simulink model "Clock_verif"  (Simulink 7.2)
settings: Solver=ode45  StartTime=0.0  StopTime=10.0  RelTol=1e-3
undefined symbols (not defined in the file): clock_sample
settings Model: Creator=Romain  LastModifiedBy=Romain
settings OptimizationCC: ExpressionDepthLimit=128
settings DebuggingCC: SolverPrmCheckMsg=none  FcnCallInpInsideContextMsg=Enable All  StateNameClashWarn=none  StrictBusMsg=ErrorLevel1
settings CodeAppCC: CustomSymbolStrType=$N$R$M_T
settings GRTTargetCC: TargetFunctionLibrary=C89/C90 (ANSI)

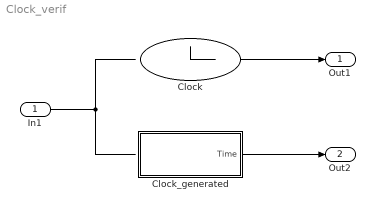
== system Clock_verif ==
  In1 : Inport  OutDataTypeStr=double  DataType=double
  Clock : Clock
  Clock_generated : Subsystem  TreatAsAtomicUnit=on
  Out1 : Outport
  Out2 : Outport  Port=2
  wires:
  In1/1 -> ?
  Clock/1 -> Out1/1
  Clock_generated/1(Time) -> Out2/1

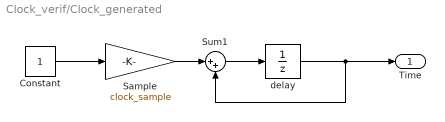
== system Clock_verif/Clock_generated ==
  Constant : Constant
  Sample : Gain  Gain=clock_sample
  Sum1 : Sum  RequirementInfo={} %GIDa_c1246c4c_805a_4e31_9fd7_94b19cd83488  Inputs=|++
  delay : UnitDelay  SampleTime=clock_sample
  Time : Outport  RequirementInfo={} %GIDa_0e000bec_2cd2_48cd_a7a7_611e17fa9ae8
  wires:
  Constant/1 -> Sample/1
  delay/1 -> Sum1/2, Time/1
  Sum1/1 -> delay/1
  Sample/1 -> Sum1/1
